simulink model "audiofilter"  (R2020b)
settings: Solver=VariableStepAuto  StartTime=0.0  StopTime=1000000  RelTol=1e-3
undefined symbols (not defined in the file): bpCoeff, hpCoeff, lpCoeff
libraries: dspsrcs4 x3, SimulinkForSyDe x1
settings Model: Creator=Andrea  LastModifiedBy=Andrea

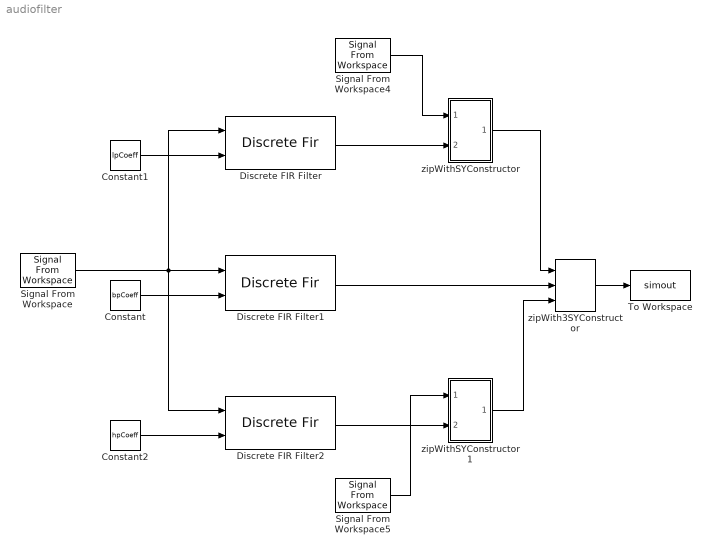
== system audiofilter ==
  Constant : Constant  Value=bpCoeff
  Constant1 : Constant  Value=lpCoeff
  Constant2 : Constant  Value=hpCoeff
  Discrete FIR Filter : DiscreteFir  CoefSource=Input port
      settings: InputPortMap=u0,u1
  Discrete FIR Filter1 : DiscreteFir  CoefSource=Input port  Coefficients=[0.0631876133978400 0.0813165121768200 0.0956232670043200 0.104783444329680 0.107936294048860 0.104783444329680 0.0956232670043200 0.0813165121768200 0.0631876133978400]
      settings: InputPortMap=u0,u1
  Discrete FIR Filter2 : DiscreteFir  CoefSource=Input port
      settings: InputPortMap=u0,u1
  Signal From Workspace : dspsrcs4/Signal From Workspace  X=audioIn  Ts=1  nsamps=1  OutputAfterFinalValue=Setting to zero  ignoreOrWarnInputAndFrameLengths=off  OutputFrames=off
  Signal From Workspace4 : dspsrcs4/Signal From Workspace  X=bass  Ts=1  nsamps=1  OutputAfterFinalValue=Setting to zero  ignoreOrWarnInputAndFrameLengths=off  OutputFrames=off
  Signal From Workspace5 : dspsrcs4/Signal From Workspace  X=treble  Ts=1  nsamps=1  OutputAfterFinalValue=Setting to zero  ignoreOrWarnInputAndFrameLengths=off  OutputFrames=off
  To Workspace : ToWorkspace  VariableName=simout  SaveFormat=Timeseries  SampleTime=-1
  zipWith3SYConstructor : SimulinkForSyDe/zipWith3SYConstructor  SystemSampleTime=-1  VariantActivationTime=update diagram  Latency=0  AutoFrameSizeCalculation=off
      settings: SourceProductName=Simulink ForSyDe
  zipWithSYConstructor : Subsystem  AncestorBlock=SimulinkForSyDe/zipWithSYConstructor
  zipWithSYConstructor1 : Subsystem  AncestorBlock=SimulinkForSyDe/zipWithSYConstructor
  wires:
  Discrete FIR Filter/1 -> zipWithSYConstructor/2(In2)
  Signal From Workspace/1 -> Discrete FIR Filter/1, Discrete FIR Filter2/1, Discrete FIR Filter1/1
  Constant2/1 -> Discrete FIR Filter2/2
  Signal From Workspace4/1 -> zipWithSYConstructor/1(In1)
  Signal From Workspace5/1 -> zipWithSYConstructor1/1(In1)
  Discrete FIR Filter2/1 -> zipWithSYConstructor1/2(In2)
  zipWithSYConstructor/1(Out1) -> zipWith3SYConstructor/1
  Discrete FIR Filter1/1 -> zipWith3SYConstructor/2
  zipWithSYConstructor1/1(Out1) -> zipWith3SYConstructor/3
  zipWith3SYConstructor/1 -> To Workspace/1
  Constant1/1 -> Discrete FIR Filter/2
  Constant/1 -> Discrete FIR Filter1/2

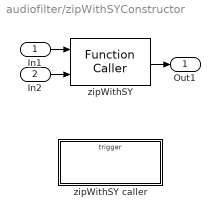
== system audiofilter/zipWithSYConstructor ==
  In1 : Inport
  In2 : Inport  Port=2
  zipWithSY : FunctionCaller  FunctionPrototype=y = zipWithSYf(u,u1)  InputArgumentSpecifications=<Enter example>  OutputArgumentSpecifications=<Enter example>
  zipWithSY caller : Subsystem  TreatAsAtomicUnit=on
  Out1 : Outport
  wires:
  In2/1 -> zipWithSY/2
  zipWithSY/1 -> Out1/1
  In1/1 -> zipWithSY/1

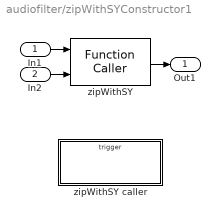
== system audiofilter/zipWithSYConstructor1 ==
  In1 : Inport
  In2 : Inport  Port=2
  zipWithSY : FunctionCaller  FunctionPrototype=y = zipWithSYf(u,u1)  InputArgumentSpecifications=<Enter example>  OutputArgumentSpecifications=<Enter example>
  zipWithSY caller : Subsystem  TreatAsAtomicUnit=on
  Out1 : Outport
  wires:
  In2/1 -> zipWithSY/2
  zipWithSY/1 -> Out1/1
  In1/1 -> zipWithSY/1

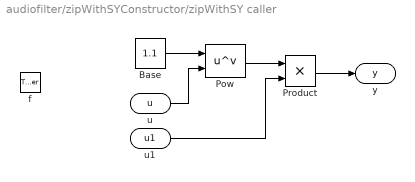
== system audiofilter/zipWithSYConstructor/zipWithSY caller ==
  f : TriggerPort  TriggerType=function-call  IsSimulinkFunction=on  FunctionName=zipWithSYf  FunctionVisibility=scoped  VariantControl=(inherit)
  Base : Constant  Value=1.1
  Pow : Math  Operator=pow  SignedPower=on  RndMeth=Zero  SaturateOnIntegerOverflow=on
  Product : Product
  u : ArgIn  DisableCoverage=on  ArgumentName=u
  u1 : ArgIn  DisableCoverage=on  Port=2  ArgumentName=u1
  y : ArgOut  DisableCoverage=on  ArgumentName=y
  wires:
  u/1 -> Pow/2
  Base/1 -> Pow/1
  Pow/1 -> Product/1
  u1/1 -> Product/2
  Product/1 -> y/1

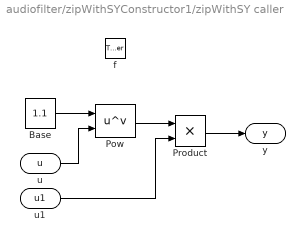
== system audiofilter/zipWithSYConstructor1/zipWithSY caller ==
  f : TriggerPort  TriggerType=function-call  IsSimulinkFunction=on  FunctionName=zipWithSYf  FunctionVisibility=scoped  VariantControl=(inherit)
  Base : Constant  Value=1.1
  Pow : Math  Operator=pow  SignedPower=on  RndMeth=Zero  SaturateOnIntegerOverflow=on
  Product : Product
  u : ArgIn  DisableCoverage=on  ArgumentName=u
  u1 : ArgIn  DisableCoverage=on  Port=2  ArgumentName=u1
  y : ArgOut  DisableCoverage=on  ArgumentName=y
  wires:
  Product/1 -> y/1
  Base/1 -> Pow/1
  Pow/1 -> Product/1
  u/1 -> Pow/2
  u1/1 -> Product/2
